simulink model "mo"  (R2015b)
settings: Solver=VariableStepAuto  StartTime=0.0  StopTime=10.0  RelTol=1e-3
settings Model: Creator=BLUE COM  LastModifiedBy=BLUE COM

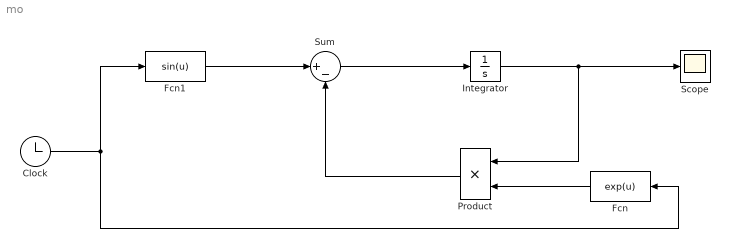
== system mo ==
  Clock : Clock
      settings: Decimation=3
  Fcn : Fcn  Expr=exp(u)
  Fcn1 : Fcn  Expr=sin(u)
  Integrator : Integrator
  Product : Product
  Scope : Scope
  Sum : Sum  Inputs=|+-
  wires:
  Integrator/1 -> Product/1, Scope/1
  Fcn/1 -> Product/2
  Sum/1 -> Integrator/1
  Product/1 -> Sum/2
  Fcn1/1 -> Sum/1
  Clock/1 -> Fcn/1, Fcn1/1
